simulink model "lookup_nD_TestGen9"  (R2017b)
settings: Solver=FixedStepDiscrete  StartTime=0.0  StopTime=10.0  RelTol=1e-3
model workspace (MAT data in the model file):
  LUTObjLKnD9 = Simulink.LookupTable
  LUTObjLKnD9.Table = Simulink.lookuptable.Table
  LUTObjLKnD9.Table.Value = [124.81870773  5.04589493667  6.12454107041  7.59264823461  41.8242865098; 103.653937611  76.950961325  100.612434313  78.8335303578  34.282883466; 24.0595124694  92.778778408  50.2007904898  20.9792672302  68.7178862504]
  LUTObjLKnD9.Table.Dimensions = [3 5]
  LUTObjLKnD9.Table.DataType = 'double'
  LUTObjLKnD9.Table.FieldName = 'Table'
  LUTObjLKnD9.Breakpoints(1) = Simulink.lookuptable.Breakpoint
  LUTObjLKnD9.Breakpoints(1).Value = [54.8907192599; 73.4084232427; 108.423218382]
  LUTObjLKnD9.Breakpoints(1).TunableSizeName = 'N1'
  LUTObjLKnD9.Breakpoints(1).Dimensions = [3 1]
  LUTObjLKnD9.Breakpoints(1).DataType = 'double'
  LUTObjLKnD9.Breakpoints(1).FieldName = 'BP1'
  LUTObjLKnD9.Breakpoints(2) = Simulink.lookuptable.Breakpoint
  LUTObjLKnD9.Breakpoints(2).Value = [17.3326893337; 73.8558281428; 80.5694174688; 85.2429361284; 106.291266458]
  LUTObjLKnD9.Breakpoints(2).TunableSizeName = 'N2'
  LUTObjLKnD9.Breakpoints(2).Dimensions = [5 1]
  LUTObjLKnD9.Breakpoints(2).DataType = 'double'
  LUTObjLKnD9.Breakpoints(2).FieldName = 'BP2'
  LUTObjLKnD9.SupportTunableSize = 0
  LUTObjLKnD9.StructTypeInfo = Simulink.lookuptable.StructTypeInfo
  LUTObjLKnD9.StructTypeInfo.Name = 'LUT'
  LUTObjLKnD9.StructTypeInfo.DataScope = 'Auto'
settings Model: Creator=ktrinh  LastModifiedBy=ktrinh
settings DebuggingCC: ParameterOverflowMsg=none

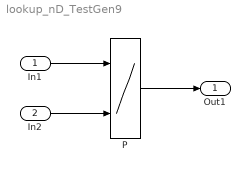
== system lookup_nD_TestGen9 ==
  In1 : Inport  OutMin=0  OutMax=127  PortDimensions=1
  In2 : Inport  Port=2  OutMin=0  OutMax=127
  P : Lookup_n-D  DataSpecification=Lookup table object  LookupTableObject=LUTObjLKnD9  BreakpointsForDimension3=[5, 7]  Table=reshape(repmat([4 5 6;16 19 20;10 18 23],1,2),[3,3,2])  InterpMethod=Nearest  ExtrapMethod=Clip  InternalRulePriority=Speed  OutDataTypeStr=double  SaturateOnIntegerOverflow=on  InputSameDT=on
  Out1 : Outport
  wires:
  In1/1 -> P/1
  In2/1 -> P/2
  P/1 -> Out1/1
